simulink model "Shanthan_Heeirthan_EE469S3D_R45 (1)"  (R2023a)
settings: Solver=FixedStepDiscrete  StartTime=0.0  StopTime=120  FixedStep=dt0  RelTol=1e-3  EnableMultiTasking=on
PostLoadFcn:
  | %Set the size for the model
  | set_param(gcs,'Location',[10 10 1270 970])
  | %Set the zoom factor for the model
  | set_param(gcs,'ZoomFactor','100')
InitFcn:
  | tic
  | % Students Add call to their M-file HERE
  | Shanthan_Heeirthan_EE460_Final
  | INIT_S3D_01
StartFcn:
  | tend0=toc;
  | tic;
StopFcn:
  | tend=toc;
  | disp(['Simulation time = ' num2str(tout(end)) ' sec'])
  | disp(['Real time = ' num2str(tend) ' sec'])
  | title('DONE')
  | SCORE=round((max(0,120-tout(end)-tend0))*4+10*(40-FuelBurned)+sum(100*double(PDONE)-100*double(PDONE<.5)));
  | PlotS3D(PlotInput);
  | text(15,22,['S: ' num2str(SCORE)]);
values from neighbouring files (symbols this model uses):
  A = [0 1 0 0 0 0 ... (first row only)    [Shanthan_Heeirthan_EE460_Final (1).m]
  B = [0 0 0 ... (first row only)    [Shanthan_Heeirthan_EE460_Final (1).m]
  bm = [1 1 -1 -1 0 0 0 0; 0 0 0 0 -1 1 1 -1; -1 1 -1 1 3 -3 3 -3]    [Shanthan_Heeirthan_EE460_Final (1).m]
  C = [1 0 0 0 0 0 ... (first row only)    [Shanthan_Heeirthan_EE460_Final (1).m]
  D = [0 0 0 ... (first row only)    [Shanthan_Heeirthan_EE460_Final (1).m]
  Denchptheta = TFchptheta.Den{1}    [Shanthan_Heeirthan_EE460_Final (1).m]
  Denchpxy = TFchpxy.Den{1}    [Shanthan_Heeirthan_EE460_Final (1).m]
  Denclptheta = TFclptheta.Den{1}    [Shanthan_Heeirthan_EE460_Final (1).m]
  Denclpxy = TFclpxy.Den{1}    [Shanthan_Heeirthan_EE460_Final (1).m]
  Denlp = TFlp.Den{1}    [Shanthan_Heeirthan_EE460_Final (1).m]
  Kd = 2.1+0    (= 2.1)    [Shanthan_Heeirthan_EE460_Final (1).m]
  Ki = 0.0001    [Shanthan_Heeirthan_EE460_Final (1).m]
  Kp = 1.1+0.2    (= 1.3)    [Shanthan_Heeirthan_EE460_Final (1).m]
  L = place(A',C',ep)'    [Shanthan_Heeirthan_EE460_Final (1).m]
  Numchptheta = TFchptheta.Num{1}    [Shanthan_Heeirthan_EE460_Final (1).m]
  Numchpxy = TFchpxy.Num{1}    [Shanthan_Heeirthan_EE460_Final (1).m]
  Numclptheta = TFclptheta.Num{1}    [Shanthan_Heeirthan_EE460_Final (1).m]
  Numclpxy = TFclpxy.Num{1}    [Shanthan_Heeirthan_EE460_Final (1).m]
  Numlp = TFlp.Num{1}    [Shanthan_Heeirthan_EE460_Final (1).m]
  Pnewdata = [LVL.P1 LVL.P2 LVL.P3 LVL.P4]    [Shanthan_Heeirthan_EE460_Final (1).m]
  Sconfig = 1    [Shanthan_Heeirthan_EE460_Final (1).m]
  TFP1 = 2    [Shanthan_Heeirthan_EE460_Final (1).m]
  TFP1z = 1    [Shanthan_Heeirthan_EE460_Final (1).m]
  TFP2 = 2    [Shanthan_Heeirthan_EE460_Final (1).m]
  TFP2z = 1    [Shanthan_Heeirthan_EE460_Final (1).m]
  TFP3 = 2    [Shanthan_Heeirthan_EE460_Final (1).m]
  TFP3z = 1    [Shanthan_Heeirthan_EE460_Final (1).m]
  TFP4 = 2    [Shanthan_Heeirthan_EE460_Final (1).m]
  TFP4z = 1    [Shanthan_Heeirthan_EE460_Final (1).m]
  wcf = 2    [Shanthan_Heeirthan_EE460_Final (1).m]
  wcft = 10    [Shanthan_Heeirthan_EE460_Final (1).m]
undefined symbols (not defined in the file or in its folder): d2r, DiscIntNeverNeededParam, dt, dt0, fr, HM_S, HM_U, J, Jbase, JC0, L13, L24, LVL, M, M1, M2, M3, M4, mdti, Pdata, PTvec, r2d, SLIM, SQ, SSF, TOLdata, ULIM
libraries: simulink x85, aerolibanimutils x1, matrix_library x1
(part 3 of 7)

== system Shanthan_Heeirthan_EE469S3D_R45 (1)/S3D_Plant/Sensors/CASE1/Yaccel ==
  X : Inport
  Abs : Abs  SaturateOnIntegerOverflow=off
  Bus Selector3 : BusSelector  OutputSignals=yddt_mps2
  CURRENT : Subsystem  TreatAsAtomicUnit=on
  Compare To Constant : simulink/Logic and Bit Operations/Compare To Constant  relop=<=  const=0.5  OutDataTypeStr=boolean
  Constant1 : Constant  Value=LVL.Sfail(6)  SampleTime=dt0
  Constant2 : Constant  Value=LVL.Sft(6,1)+rand*(LVL.Sft(6,2)-LVL.Sft(6,1))  SampleTime=dt0
  Digital Clock : DigitalClock  SampleTime=dt0
  Gain : Gain  Gain=LVL.SN
  If : If  IfExpression=u1 < -0.5  ElseIfExpressions=u1 > 0.5 & u1 < 1.5
  Logical Operator : Logic  Operator=OR  AllPortsSameDT=off  OutDataTypeStr=boolean
  MAX : Subsystem  TreatAsAtomicUnit=on
  MIN : Subsystem  TreatAsAtomicUnit=on
  Merge : Merge  Inputs=3
  Quantizer : Quantizer  QuantizationInterval=SQ(6)  SampleTime=dt0
  Random Number : RandomNumber  Variance=LVL.SigSense(6)  Seed=6  SampleTime=dt0
  Relational Operator : RelationalOperator  Operator=<  OutDataTypeStr=boolean  InputSameDT=off
  Saturation : Saturate  UpperLimit=SLIM(6,2)  LowerLimit=SLIM(6,1)
  Sum : Sum  Inputs=|++
  Switch : Switch  Criteria=u2 > Threshold  SaturateOnIntegerOverflow=off  InputSameDT=off
  Unit Delay : UnitDelay  SampleTime=dt0  HasFrameUpgradeWarning=on
  yddt1 : Outport
  wires:
  Saturation/1 -> Quantizer/1
  Quantizer/1 -> yddt1/1, Unit Delay/1
  If/1 -> MIN/Action
  If/2 -> MAX/Action
  Switch/1 -> Saturation/1
  Digital Clock/1 -> Relational Operator/1
  If/3 -> CURRENT/Action
  Unit Delay/1 -> CURRENT/1(In1)
  MAX/1(Out1) -> Merge/2
  Constant2/1 -> Relational Operator/2
  X/1 -> Bus Selector3/1
  CURRENT/1(Out1) -> Merge/3
  MIN/1(Out1) -> Merge/1
  Merge/1 -> Switch/3
  Random Number/1 -> Gain/1
  Gain/1 -> Sum/2
  Bus Selector3/1 -> Sum/1  "<yddt_mps2>"
  Sum/1 -> Switch/1
  Relational Operator/1 -> Logical Operator/1
  Logical Operator/1 -> Switch/2
  Constant1/1 -> Abs/1, If/1
  Abs/1 -> Compare To Constant/1
  Compare To Constant/1 -> Logical Operator/2

== system Shanthan_Heeirthan_EE469S3D_R45 (1)/S3D_Plant/Sensors/CASE1/Ypos1 ==
  X : Inport
  Abs : Abs  SaturateOnIntegerOverflow=off
  Bus Selector3 : BusSelector  OutputSignals=y_m
  CURRENT : Subsystem  TreatAsAtomicUnit=on
  Compare To Constant : simulink/Logic and Bit Operations/Compare To Constant  relop=<=  const=0.5  OutDataTypeStr=boolean
  Constant1 : Constant  Value=LVL.Sfail(4)  SampleTime=dt0
  Constant2 : Constant  Value=LVL.Sft(4,1)+rand*(LVL.Sft(4,2)-LVL.Sft(4,1))  SampleTime=dt0
  Digital Clock : DigitalClock  SampleTime=dt0
  Gain : Gain  Gain=LVL.SN
  If : If  IfExpression=u1 < -0.5  ElseIfExpressions=u1 > 0.5 & u1 < 1.5
  Logical Operator : Logic  Operator=OR  AllPortsSameDT=off  OutDataTypeStr=boolean
  MAX : Subsystem  TreatAsAtomicUnit=on
  MIN : Subsystem  TreatAsAtomicUnit=on
  Merge : Merge  Inputs=3
  Quantizer : Quantizer  QuantizationInterval=SQ(4)  SampleTime=dt0
  Random Number : RandomNumber  Variance=LVL.SigSense(4)  Seed=4  SampleTime=dt0
  Relational Operator : RelationalOperator  Operator=<  OutDataTypeStr=boolean  InputSameDT=off
  Saturation : Saturate  UpperLimit=SLIM(4,2)  LowerLimit=SLIM(4,1)
  Sum : Sum  Inputs=|++
  Switch : Switch  Criteria=u2 > Threshold  SaturateOnIntegerOverflow=off  InputSameDT=off
  Unit Delay : UnitDelay  SampleTime=dt0  HasFrameUpgradeWarning=on
  y1 : Outport
  wires:
  Saturation/1 -> Quantizer/1
  Quantizer/1 -> y1/1, Unit Delay/1
  If/1 -> MIN/Action
  If/2 -> MAX/Action
  Switch/1 -> Saturation/1
  Digital Clock/1 -> Relational Operator/1
  If/3 -> CURRENT/Action
  Unit Delay/1 -> CURRENT/1(In1)
  MAX/1(Out1) -> Merge/2
  Constant2/1 -> Relational Operator/2
  X/1 -> Bus Selector3/1
  CURRENT/1(Out1) -> Merge/3
  MIN/1(Out1) -> Merge/1
  Merge/1 -> Switch/3
  Random Number/1 -> Gain/1
  Gain/1 -> Sum/2
  Bus Selector3/1 -> Sum/1  "<y_m>"
  Sum/1 -> Switch/1
  Relational Operator/1 -> Logical Operator/1
  Logical Operator/1 -> Switch/2
  Constant1/1 -> Abs/1, If/1
  Abs/1 -> Compare To Constant/1
  Compare To Constant/1 -> Logical Operator/2

== system Shanthan_Heeirthan_EE469S3D_R45 (1)/S3D_Plant/Sensors/CASE1/Yvel ==
  X : Inport
  Abs : Abs  SaturateOnIntegerOverflow=off
  Bus Selector3 : BusSelector  OutputSignals=ydt_mps
  CURRENT : Subsystem  TreatAsAtomicUnit=on
  Compare To Constant : simulink/Logic and Bit Operations/Compare To Constant  relop=<=  const=0.5  OutDataTypeStr=boolean
  Constant1 : Constant  Value=LVL.Sfail(5)  SampleTime=dt0
  Constant2 : Constant  Value=LVL.Sft(5,1)+rand*(LVL.Sft(5,2)-LVL.Sft(5,1))  SampleTime=dt0
  Digital Clock : DigitalClock  SampleTime=dt0
  Gain : Gain  Gain=LVL.SN
  If : If  IfExpression=u1 < -0.5  ElseIfExpressions=u1 > 0.5 & u1 < 1.5
  Logical Operator : Logic  Operator=OR  AllPortsSameDT=off  OutDataTypeStr=boolean
  MAX : Subsystem  TreatAsAtomicUnit=on
  MIN : Subsystem  TreatAsAtomicUnit=on
  Merge : Merge  Inputs=3
  Quantizer : Quantizer  QuantizationInterval=SQ(5)  SampleTime=dt0
  Random Number : RandomNumber  Variance=LVL.SigSense(5)  Seed=5  SampleTime=dt0
  Relational Operator : RelationalOperator  Operator=<  OutDataTypeStr=boolean  InputSameDT=off
  Saturation : Saturate  UpperLimit=SLIM(5,2)  LowerLimit=SLIM(5,1)
  Sum : Sum  Inputs=|++
  Switch : Switch  Criteria=u2 > Threshold  SaturateOnIntegerOverflow=off  InputSameDT=off
  Unit Delay : UnitDelay  SampleTime=dt0  HasFrameUpgradeWarning=on
  ydt1 : Outport
  wires:
  Saturation/1 -> Quantizer/1
  Quantizer/1 -> Unit Delay/1, ydt1/1
  Compare To Constant/1 -> Logical Operator/2
  Abs/1 -> Compare To Constant/1
  Constant1/1 -> If/1, Abs/1
  Logical Operator/1 -> Switch/2
  Relational Operator/1 -> Logical Operator/1
  Sum/1 -> Switch/1
  Bus Selector3/1 -> Sum/1  "<ydt_mps>"
  Gain/1 -> Sum/2
  Random Number/1 -> Gain/1
  Merge/1 -> Switch/3
  MIN/1(Out1) -> Merge/1
  CURRENT/1(Out1) -> Merge/3
  X/1 -> Bus Selector3/1
  Constant2/1 -> Relational Operator/2
  MAX/1(Out1) -> Merge/2
  Unit Delay/1 -> CURRENT/1(In1)
  If/3 -> CURRENT/Action
  Digital Clock/1 -> Relational Operator/1
  Switch/1 -> Saturation/1
  If/2 -> MAX/Action
  If/1 -> MIN/Action

== system Shanthan_Heeirthan_EE469S3D_R45 (1)/S3D_Plant/Sensors/CASE2/THTpos1 ==
  X : Inport
  Abs : Abs  SaturateOnIntegerOverflow=off
  Bus Selector3 : BusSelector  OutputSignals=tht_rad
  CURRENT : Subsystem  TreatAsAtomicUnit=on
  Compare To Constant : simulink/Logic and Bit Operations/Compare To Constant  relop=<=  const=0.5  OutDataTypeStr=boolean
  Constant1 : Constant  Value=LVL.Sfail(7)  SampleTime=dt0
  Constant2 : Constant  Value=LVL.Sft(7,1)+rand*(LVL.Sft(7,2)-LVL.Sft(7,1))  SampleTime=dt0
  Digital Clock : DigitalClock  SampleTime=dt0
  Gain : Gain  Gain=LVL.SN
  Gain4 : Gain  Gain=r2d
  If : If  IfExpression=u1 < -0.5  ElseIfExpressions=u1 > 0.5 & u1 < 1.5
  Logical Operator : Logic  Operator=OR  AllPortsSameDT=off  OutDataTypeStr=boolean
  MAX : Subsystem  TreatAsAtomicUnit=on
  MIN : Subsystem  TreatAsAtomicUnit=on
  Merge : Merge  Inputs=3
  Quantizer : Quantizer  QuantizationInterval=SQ(7)  SampleTime=dt0
  Random Number : RandomNumber  Variance=LVL.SigSense(7)  Seed=7  SampleTime=dt0
  Relational Operator : RelationalOperator  Operator=<  OutDataTypeStr=boolean  InputSameDT=off
  Saturation : Saturate  UpperLimit=SLIM(7,2)  LowerLimit=SLIM(7,1)
  Sum : Sum  Inputs=|++
  Switch : Switch  Criteria=u2 > Threshold  SaturateOnIntegerOverflow=off  InputSameDT=off
  Unit Delay : UnitDelay  SampleTime=dt0  HasFrameUpgradeWarning=on
  tht1 : Outport
  wires:
  Saturation/1 -> Quantizer/1
  Switch/1 -> Saturation/1
  If/1 -> MIN/Action
  If/2 -> MAX/Action
  Digital Clock/1 -> Relational Operator/1
  If/3 -> CURRENT/Action
  Unit Delay/1 -> CURRENT/1(In1)
  MAX/1(Out1) -> Merge/2
  Constant2/1 -> Relational Operator/2
  X/1 -> Bus Selector3/1
  CURRENT/1(Out1) -> Merge/3
  MIN/1(Out1) -> Merge/1
  Merge/1 -> Switch/3
  Random Number/1 -> Gain/1
  Gain/1 -> Sum/2
  Bus Selector3/1 -> Gain4/1  "<tht_rad>"
  Sum/1 -> Switch/1
  Relational Operator/1 -> Logical Operator/1
  Logical Operator/1 -> Switch/2
  Constant1/1 -> Abs/1, If/1
  Abs/1 -> Compare To Constant/1
  Compare To Constant/1 -> Logical Operator/2
  Gain4/1 -> Sum/1
  Quantizer/1 -> Unit Delay/1, tht1/1

== system Shanthan_Heeirthan_EE469S3D_R45 (1)/S3D_Plant/Sensors/CASE2/THTpos2 ==
  X : Inport
  Abs : Abs  SaturateOnIntegerOverflow=off
  Bus Selector3 : BusSelector  OutputSignals=tht_rad
  CURRENT : Subsystem  TreatAsAtomicUnit=on
  Compare To Constant : simulink/Logic and Bit Operations/Compare To Constant  relop=<=  const=0.5  OutDataTypeStr=boolean
  Constant1 : Constant  Value=LVL.Sfail(8)  SampleTime=dt0
  Constant2 : Constant  Value=LVL.Sft(8,1)+rand*(LVL.Sft(8,2)-LVL.Sft(8,1))  SampleTime=dt0
  Digital Clock : DigitalClock  SampleTime=dt0
  Gain : Gain  Gain=LVL.SN
  Gain4 : Gain  Gain=r2d
  If : If  IfExpression=u1 < -0.5  ElseIfExpressions=u1 > 0.5 & u1 < 1.5
  Logical Operator : Logic  Operator=OR  AllPortsSameDT=off  OutDataTypeStr=boolean
  MAX : Subsystem  TreatAsAtomicUnit=on
  MIN : Subsystem  TreatAsAtomicUnit=on
  Merge : Merge  Inputs=3
  Quantizer : Quantizer  QuantizationInterval=SQ(7)  SampleTime=dt0
  Random Number : RandomNumber  Variance=LVL.SigSense(7)  Seed=8  SampleTime=dt0
  Relational Operator : RelationalOperator  Operator=<  OutDataTypeStr=boolean  InputSameDT=off
  Saturation : Saturate  UpperLimit=SLIM(7,2)  LowerLimit=SLIM(7,1)
  Sum : Sum  Inputs=|++
  Switch : Switch  Criteria=u2 > Threshold  SaturateOnIntegerOverflow=off  InputSameDT=off
  Unit Delay : UnitDelay  SampleTime=dt0  HasFrameUpgradeWarning=on
  tht1 : Outport
  wires:
  Saturation/1 -> Quantizer/1
  Switch/1 -> Saturation/1
  Quantizer/1 -> Unit Delay/1, tht1/1
  Gain4/1 -> Sum/1
  Compare To Constant/1 -> Logical Operator/2
  Abs/1 -> Compare To Constant/1
  Constant1/1 -> If/1, Abs/1
  Logical Operator/1 -> Switch/2
  Relational Operator/1 -> Logical Operator/1
  Sum/1 -> Switch/1
  Bus Selector3/1 -> Gain4/1  "<tht_rad>"
  Gain/1 -> Sum/2
  Random Number/1 -> Gain/1
  Merge/1 -> Switch/3
  MIN/1(Out1) -> Merge/1
  CURRENT/1(Out1) -> Merge/3
  X/1 -> Bus Selector3/1
  Constant2/1 -> Relational Operator/2
  MAX/1(Out1) -> Merge/2
  Unit Delay/1 -> CURRENT/1(In1)
  If/3 -> CURRENT/Action
  Digital Clock/1 -> Relational Operator/1
  If/2 -> MAX/Action
  If/1 -> MIN/Action

== system Shanthan_Heeirthan_EE469S3D_R45 (1)/S3D_Plant/Sensors/CASE2/THTvel ==
  X : Inport
  Abs : Abs  SaturateOnIntegerOverflow=off
  Bus Selector3 : BusSelector  OutputSignals=thtdt_rps
  CURRENT : Subsystem  TreatAsAtomicUnit=on
  Compare To Constant : simulink/Logic and Bit Operations/Compare To Constant  relop=<=  const=0.5  OutDataTypeStr=boolean
  Constant1 : Constant  Value=LVL.Sfail(9)  SampleTime=dt0
  Constant2 : Constant  Value=LVL.Sft(9,1)+rand*(LVL.Sft(9,2)-LVL.Sft(9,1))  SampleTime=dt0
  Digital Clock : DigitalClock  SampleTime=dt0
  Gain : Gain  Gain=LVL.SN
  Gain4 : Gain  Gain=r2d
  If : If  IfExpression=u1 < -0.5  ElseIfExpressions=u1 > 0.5 & u1 < 1.5
  Logical Operator : Logic  Operator=OR  AllPortsSameDT=off  OutDataTypeStr=boolean
  MAX : Subsystem  TreatAsAtomicUnit=on
  MIN : Subsystem  TreatAsAtomicUnit=on
  Merge : Merge  Inputs=3
  Quantizer : Quantizer  QuantizationInterval=SQ(8)  SampleTime=dt0
  Random Number : RandomNumber  Variance=LVL.SigSense(8)  Seed=9  SampleTime=dt0
  Relational Operator : RelationalOperator  Operator=<  OutDataTypeStr=boolean  InputSameDT=off
  Saturation : Saturate  UpperLimit=SLIM(8,2)  LowerLimit=SLIM(8,1)
  Sum : Sum  Inputs=|++
  Switch : Switch  Criteria=u2 > Threshold  SaturateOnIntegerOverflow=off  InputSameDT=off
  Unit Delay : UnitDelay  SampleTime=dt0  HasFrameUpgradeWarning=on
  thtdt1 : Outport
  wires:
  Saturation/1 -> Quantizer/1
  Compare To Constant/1 -> Logical Operator/2
  Abs/1 -> Compare To Constant/1
  Constant1/1 -> If/1, Abs/1
  Logical Operator/1 -> Switch/2
  Relational Operator/1 -> Logical Operator/1
  Sum/1 -> Switch/1
  Bus Selector3/1 -> Gain4/1  "<thtdt_rps>"
  Gain/1 -> Sum/2
  Random Number/1 -> Gain/1
  Merge/1 -> Switch/3
  MIN/1(Out1) -> Merge/1
  CURRENT/1(Out1) -> Merge/3
  X/1 -> Bus Selector3/1
  Constant2/1 -> Relational Operator/2
  MAX/1(Out1) -> Merge/2
  Unit Delay/1 -> CURRENT/1(In1)
  If/3 -> CURRENT/Action
  Digital Clock/1 -> Relational Operator/1
  Switch/1 -> Saturation/1
  If/2 -> MAX/Action
  If/1 -> MIN/Action
  Gain4/1 -> Sum/1
  Quantizer/1 -> Unit Delay/1, thtdt1/1

== system Shanthan_Heeirthan_EE469S3D_R45 (1)/S3D_Plant/Sensors/CASE2/Xpos1 ==
  X : Inport
  Abs : Abs  SaturateOnIntegerOverflow=off
  Bus Selector3 : BusSelector  OutputSignals=x_m
  CURRENT : Subsystem  TreatAsAtomicUnit=on
  Compare To Constant : simulink/Logic and Bit Operations/Compare To Constant  relop=<=  const=0.5  OutDataTypeStr=boolean
  Constant1 : Constant  Value=LVL.Sfail(1)  SampleTime=dt0
  Constant2 : Constant  Value=LVL.Sft(1,1)+rand*(LVL.Sft(1,2)-LVL.Sft(1,1))  SampleTime=dt0
  Digital Clock : DigitalClock  SampleTime=dt0
  Gain : Gain  Gain=LVL.SN
  If : If  IfExpression=u1 < -0.5  ElseIfExpressions=u1 > 0.5 & u1 < 1.5
  Logical Operator : Logic  Operator=OR  AllPortsSameDT=off  OutDataTypeStr=boolean
  MAX : Subsystem  TreatAsAtomicUnit=on
  MIN : Subsystem  TreatAsAtomicUnit=on
  Merge : Merge  Inputs=3
  Quantizer : Quantizer  QuantizationInterval=SQ(1)  SampleTime=dt0
  Random Number : RandomNumber  Variance=LVL.SigSense(1)  Seed=1  SampleTime=dt0
  Relational Operator : RelationalOperator  Operator=<  OutDataTypeStr=boolean  InputSameDT=off
  Saturation : Saturate  UpperLimit=SLIM(1,2)  LowerLimit=SLIM(1,1)
  Sum : Sum  Inputs=|++
  Switch : Switch  Criteria=u2 > Threshold  SaturateOnIntegerOverflow=off  InputSameDT=off
  Unit Delay : UnitDelay  SampleTime=dt0  HasFrameUpgradeWarning=on
  x1 : Outport
  wires:
  Saturation/1 -> Quantizer/1
  If/1 -> MIN/Action
  If/2 -> MAX/Action
  Switch/1 -> Saturation/1
  Digital Clock/1 -> Relational Operator/1
  If/3 -> CURRENT/Action
  Unit Delay/1 -> CURRENT/1(In1)
  MAX/1(Out1) -> Merge/2
  Constant2/1 -> Relational Operator/2
  X/1 -> Bus Selector3/1
  CURRENT/1(Out1) -> Merge/3
  MIN/1(Out1) -> Merge/1
  Merge/1 -> Switch/3
  Random Number/1 -> Gain/1
  Gain/1 -> Sum/2
  Bus Selector3/1 -> Sum/1  "<x_m>"
  Sum/1 -> Switch/1
  Relational Operator/1 -> Logical Operator/1
  Logical Operator/1 -> Switch/2
  Constant1/1 -> Abs/1, If/1
  Abs/1 -> Compare To Constant/1
  Compare To Constant/1 -> Logical Operator/2
  Quantizer/1 -> x1/1, Unit Delay/1

== system Shanthan_Heeirthan_EE469S3D_R45 (1)/S3D_Plant/Sensors/CASE2/Xpos2 ==
  X : Inport
  Abs : Abs  SaturateOnIntegerOverflow=off
  Bus Selector3 : BusSelector  OutputSignals=x_m
  CURRENT : Subsystem  TreatAsAtomicUnit=on
  Compare To Constant : simulink/Logic and Bit Operations/Compare To Constant  relop=<=  const=0.5  OutDataTypeStr=boolean
  Constant1 : Constant  Value=LVL.Sfail(2)  SampleTime=dt0
  Constant2 : Constant  Value=LVL.Sft(2,1)+rand*(LVL.Sft(2,2)-LVL.Sft(2,1))  SampleTime=dt0
  Digital Clock : DigitalClock  SampleTime=dt0
  Gain : Gain  Gain=LVL.SN
  If : If  IfExpression=u1 < -0.5  ElseIfExpressions=u1 > 0.5 & u1 < 1.5
  Logical Operator : Logic  Operator=OR  AllPortsSameDT=off  OutDataTypeStr=boolean
  MAX : Subsystem  TreatAsAtomicUnit=on
  MIN : Subsystem  TreatAsAtomicUnit=on
  Merge : Merge  Inputs=3
  Quantizer : Quantizer  QuantizationInterval=SQ(1)  SampleTime=dt0
  Random Number : RandomNumber  Variance=LVL.SigSense(1)  Seed=2  SampleTime=dt0
  Relational Operator : RelationalOperator  Operator=<  OutDataTypeStr=boolean  InputSameDT=off
  Saturation : Saturate  UpperLimit=SLIM(1,2)  LowerLimit=SLIM(1,1)
  Sum : Sum  Inputs=|++
  Switch : Switch  Criteria=u2 > Threshold  SaturateOnIntegerOverflow=off  InputSameDT=off
  Unit Delay : UnitDelay  SampleTime=dt0  HasFrameUpgradeWarning=on
  x1 : Outport
  wires:
  Saturation/1 -> Quantizer/1
  Quantizer/1 -> Unit Delay/1, x1/1
  Compare To Constant/1 -> Logical Operator/2
  Abs/1 -> Compare To Constant/1
  Constant1/1 -> If/1, Abs/1
  Logical Operator/1 -> Switch/2
  Relational Operator/1 -> Logical Operator/1
  Sum/1 -> Switch/1
  Bus Selector3/1 -> Sum/1  "<x_m>"
  Gain/1 -> Sum/2
  Random Number/1 -> Gain/1
  Merge/1 -> Switch/3
  MIN/1(Out1) -> Merge/1
  CURRENT/1(Out1) -> Merge/3
  X/1 -> Bus Selector3/1
  Constant2/1 -> Relational Operator/2
  MAX/1(Out1) -> Merge/2
  Unit Delay/1 -> CURRENT/1(In1)
  If/3 -> CURRENT/Action
  Digital Clock/1 -> Relational Operator/1
  Switch/1 -> Saturation/1
  If/2 -> MAX/Action
  If/1 -> MIN/Action

== system Shanthan_Heeirthan_EE469S3D_R45 (1)/S3D_Plant/Sensors/CASE2/Xvel ==
  X : Inport
  Abs : Abs  SaturateOnIntegerOverflow=off
  Bus Selector3 : BusSelector  OutputSignals=xdt_mps
  CURRENT : Subsystem  TreatAsAtomicUnit=on
  Compare To Constant : simulink/Logic and Bit Operations/Compare To Constant  relop=<=  const=0.5  OutDataTypeStr=boolean
  Constant1 : Constant  Value=LVL.Sfail(3)  SampleTime=dt0
  Constant2 : Constant  Value=LVL.Sft(3,1)+rand*(LVL.Sft(3,2)-LVL.Sft(3,1))  SampleTime=dt0
  Digital Clock : DigitalClock  SampleTime=dt0
  Gain : Gain  Gain=LVL.SN
  If : If  IfExpression=u1 < -0.5  ElseIfExpressions=u1 > 0.5 & u1 < 1.5
  Logical Operator : Logic  Operator=OR  AllPortsSameDT=off  OutDataTypeStr=boolean
  MAX : Subsystem  TreatAsAtomicUnit=on
  MIN : Subsystem  TreatAsAtomicUnit=on
  Merge : Merge  Inputs=3
  Quantizer : Quantizer  QuantizationInterval=SQ(2)  SampleTime=dt0
  Random Number : RandomNumber  Variance=LVL.SigSense(2)  Seed=3  SampleTime=dt0
  Relational Operator : RelationalOperator  Operator=<  OutDataTypeStr=boolean  InputSameDT=off
  Saturation : Saturate  UpperLimit=SLIM(2,2)  LowerLimit=SLIM(2,1)
  Sum : Sum  Inputs=|++
  Switch : Switch  Criteria=u2 > Threshold  SaturateOnIntegerOverflow=off  InputSameDT=off
  Unit Delay : UnitDelay  SampleTime=dt0  HasFrameUpgradeWarning=on
  xdt1 : Outport
  wires:
  Saturation/1 -> Quantizer/1
  Compare To Constant/1 -> Logical Operator/2
  Abs/1 -> Compare To Constant/1
  Constant1/1 -> If/1, Abs/1
  Logical Operator/1 -> Switch/2
  Relational Operator/1 -> Logical Operator/1
  Sum/1 -> Switch/1
  Bus Selector3/1 -> Sum/1  "<xdt_mps>"
  Gain/1 -> Sum/2
  Random Number/1 -> Gain/1
  Merge/1 -> Switch/3
  MIN/1(Out1) -> Merge/1
  CURRENT/1(Out1) -> Merge/3
  X/1 -> Bus Selector3/1
  Constant2/1 -> Relational Operator/2
  MAX/1(Out1) -> Merge/2
  Unit Delay/1 -> CURRENT/1(In1)
  If/3 -> CURRENT/Action
  Digital Clock/1 -> Relational Operator/1
  Switch/1 -> Saturation/1
  If/2 -> MAX/Action
  If/1 -> MIN/Action
  Quantizer/1 -> Unit Delay/1, xdt1/1

== system Shanthan_Heeirthan_EE469S3D_R45 (1)/S3D_Plant/Sensors/CASE2/Ypos1 ==
  X : Inport
  Abs : Abs  SaturateOnIntegerOverflow=off
  Bus Selector3 : BusSelector  OutputSignals=y_m
  CURRENT : Subsystem  TreatAsAtomicUnit=on
  Compare To Constant : simulink/Logic and Bit Operations/Compare To Constant  relop=<=  const=0.5  OutDataTypeStr=boolean
  Constant1 : Constant  Value=LVL.Sfail(4)  SampleTime=dt0
  Constant2 : Constant  Value=LVL.Sft(4,1)+rand*(LVL.Sft(4,2)-LVL.Sft(4,1))  SampleTime=dt0
  Digital Clock : DigitalClock  SampleTime=dt0
  Gain : Gain  Gain=LVL.SN
  If : If  IfExpression=u1 < -0.5  ElseIfExpressions=u1 > 0.5 & u1 < 1.5
  Logical Operator : Logic  Operator=OR  AllPortsSameDT=off  OutDataTypeStr=boolean
  MAX : Subsystem  TreatAsAtomicUnit=on
  MIN : Subsystem  TreatAsAtomicUnit=on
  Merge : Merge  Inputs=3
  Quantizer : Quantizer  QuantizationInterval=SQ(4)  SampleTime=dt0
  Random Number : RandomNumber  Variance=LVL.SigSense(4)  Seed=4  SampleTime=dt0
  Relational Operator : RelationalOperator  Operator=<  OutDataTypeStr=boolean  InputSameDT=off
  Saturation : Saturate  UpperLimit=SLIM(4,2)  LowerLimit=SLIM(4,1)
  Sum : Sum  Inputs=|++
  Switch : Switch  Criteria=u2 > Threshold  SaturateOnIntegerOverflow=off  InputSameDT=off
  Unit Delay : UnitDelay  SampleTime=dt0  HasFrameUpgradeWarning=on
  y1 : Outport
  wires:
  Saturation/1 -> Quantizer/1
  Compare To Constant/1 -> Logical Operator/2
  Abs/1 -> Compare To Constant/1
  Constant1/1 -> If/1, Abs/1
  Logical Operator/1 -> Switch/2
  Relational Operator/1 -> Logical Operator/1
  Sum/1 -> Switch/1
  Bus Selector3/1 -> Sum/1  "<y_m>"
  Gain/1 -> Sum/2
  Random Number/1 -> Gain/1
  Merge/1 -> Switch/3
  MIN/1(Out1) -> Merge/1
  CURRENT/1(Out1) -> Merge/3
  X/1 -> Bus Selector3/1
  Constant2/1 -> Relational Operator/2
  MAX/1(Out1) -> Merge/2
  Unit Delay/1 -> CURRENT/1(In1)
  If/3 -> CURRENT/Action
  Digital Clock/1 -> Relational Operator/1
  Switch/1 -> Saturation/1
  If/2 -> MAX/Action
  If/1 -> MIN/Action
  Quantizer/1 -> Unit Delay/1, y1/1

== system Shanthan_Heeirthan_EE469S3D_R45 (1)/S3D_Plant/Sensors/CASE2/Ypos2 ==
  X : Inport
  Abs : Abs  SaturateOnIntegerOverflow=off
  Bus Selector3 : BusSelector  OutputSignals=y_m
  CURRENT : Subsystem  TreatAsAtomicUnit=on
  Compare To Constant : simulink/Logic and Bit Operations/Compare To Constant  relop=<=  const=0.5  OutDataTypeStr=boolean
  Constant1 : Constant  Value=LVL.Sfail(5)  SampleTime=dt0
  Constant2 : Constant  Value=LVL.Sft(5,1)+rand*(LVL.Sft(5,2)-LVL.Sft(5,1))  SampleTime=dt0
  Digital Clock : DigitalClock  SampleTime=dt0
  Gain : Gain  Gain=LVL.SN
  If : If  IfExpression=u1 < -0.5  ElseIfExpressions=u1 > 0.5 & u1 < 1.5
  Logical Operator : Logic  Operator=OR  AllPortsSameDT=off  OutDataTypeStr=boolean
  MAX : Subsystem  TreatAsAtomicUnit=on
  MIN : Subsystem  TreatAsAtomicUnit=on
  Merge : Merge  Inputs=3
  Quantizer : Quantizer  QuantizationInterval=SQ(4)  SampleTime=dt0
  Random Number : RandomNumber  Variance=LVL.SigSense(4)  Seed=5  SampleTime=dt0
  Relational Operator : RelationalOperator  Operator=<  OutDataTypeStr=boolean  InputSameDT=off
  Saturation : Saturate  UpperLimit=SLIM(4,2)  LowerLimit=SLIM(4,1)
  Sum : Sum  Inputs=|++
  Switch : Switch  Criteria=u2 > Threshold  SaturateOnIntegerOverflow=off  InputSameDT=off
  Unit Delay : UnitDelay  SampleTime=dt0  HasFrameUpgradeWarning=on
  y1 : Outport
  wires:
  Saturation/1 -> Quantizer/1
  Quantizer/1 -> y1/1, Unit Delay/1
  If/1 -> MIN/Action
  If/2 -> MAX/Action
  Switch/1 -> Saturation/1
  Digital Clock/1 -> Relational Operator/1
  If/3 -> CURRENT/Action
  Unit Delay/1 -> CURRENT/1(In1)
  MAX/1(Out1) -> Merge/2
  Constant2/1 -> Relational Operator/2
  X/1 -> Bus Selector3/1
  CURRENT/1(Out1) -> Merge/3
  MIN/1(Out1) -> Merge/1
  Merge/1 -> Switch/3
  Random Number/1 -> Gain/1
  Gain/1 -> Sum/2
  Bus Selector3/1 -> Sum/1  "<y_m>"
  Sum/1 -> Switch/1
  Relational Operator/1 -> Logical Operator/1
  Logical Operator/1 -> Switch/2
  Constant1/1 -> Abs/1, If/1
  Abs/1 -> Compare To Constant/1
  Compare To Constant/1 -> Logical Operator/2

== system Shanthan_Heeirthan_EE469S3D_R45 (1)/S3D_Plant/Sensors/CASE2/Yvel ==
  X : Inport
  Abs : Abs  SaturateOnIntegerOverflow=off
  Bus Selector3 : BusSelector  OutputSignals=ydt_mps
  CURRENT : Subsystem  TreatAsAtomicUnit=on
  Compare To Constant : simulink/Logic and Bit Operations/Compare To Constant  relop=<=  const=0.5  OutDataTypeStr=boolean
  Constant1 : Constant  Value=LVL.Sfail(6)  SampleTime=dt0
  Constant2 : Constant  Value=LVL.Sft(6,1)+rand*(LVL.Sft(6,2)-LVL.Sft(6,1))  SampleTime=dt0
  Digital Clock : DigitalClock  SampleTime=dt0
  Gain : Gain  Gain=LVL.SN
  If : If  IfExpression=u1 < -0.5  ElseIfExpressions=u1 > 0.5 & u1 < 1.5
  Logical Operator : Logic  Operator=OR  AllPortsSameDT=off  OutDataTypeStr=boolean
  MAX : Subsystem  TreatAsAtomicUnit=on
  MIN : Subsystem  TreatAsAtomicUnit=on
  Merge : Merge  Inputs=3
  Quantizer : Quantizer  QuantizationInterval=SQ(5)  SampleTime=dt0
  Random Number : RandomNumber  Variance=LVL.SigSense(5)  Seed=6  SampleTime=dt0
  Relational Operator : RelationalOperator  Operator=<  OutDataTypeStr=boolean  InputSameDT=off
  Saturation : Saturate  UpperLimit=SLIM(5,2)  LowerLimit=SLIM(5,1)
  Sum : Sum  Inputs=|++
  Switch : Switch  Criteria=u2 > Threshold  SaturateOnIntegerOverflow=off  InputSameDT=off
  Unit Delay : UnitDelay  SampleTime=dt0  HasFrameUpgradeWarning=on
  ydt1 : Outport
  wires:
  Saturation/1 -> Quantizer/1
  If/1 -> MIN/Action
  If/2 -> MAX/Action
  Switch/1 -> Saturation/1
  Digital Clock/1 -> Relational Operator/1
  If/3 -> CURRENT/Action
  Unit Delay/1 -> CURRENT/1(In1)
  MAX/1(Out1) -> Merge/2
  Constant2/1 -> Relational Operator/2
  X/1 -> Bus Selector3/1
  CURRENT/1(Out1) -> Merge/3
  MIN/1(Out1) -> Merge/1
  Merge/1 -> Switch/3
  Random Number/1 -> Gain/1
  Gain/1 -> Sum/2
  Bus Selector3/1 -> Sum/1  "<ydt_mps>"
  Sum/1 -> Switch/1
  Relational Operator/1 -> Logical Operator/1
  Logical Operator/1 -> Switch/2
  Constant1/1 -> Abs/1, If/1
  Abs/1 -> Compare To Constant/1
  Compare To Constant/1 -> Logical Operator/2
  Quantizer/1 -> ydt1/1, Unit Delay/1

== system Shanthan_Heeirthan_EE469S3D_R45 (1)/S3D_Plant/Sensors/CASE3/THTpos1 ==
  X : Inport
  Abs : Abs  SaturateOnIntegerOverflow=off
  Bus Selector3 : BusSelector  OutputSignals=tht_rad
  CURRENT : Subsystem  TreatAsAtomicUnit=on
  Compare To Constant : simulink/Logic and Bit Operations/Compare To Constant  relop=<=  const=0.5  OutDataTypeStr=boolean
  Constant1 : Constant  Value=LVL.Sfail(7)  SampleTime=dt0
  Constant2 : Constant  Value=LVL.Sft(7,1)+rand*(LVL.Sft(7,2)-LVL.Sft(7,1))  SampleTime=dt0
  Digital Clock : DigitalClock  SampleTime=dt0
  Gain : Gain  Gain=LVL.SN
  Gain4 : Gain  Gain=r2d
  If : If  IfExpression=u1 < -0.5  ElseIfExpressions=u1 > 0.5 & u1 < 1.5
  Logical Operator : Logic  Operator=OR  AllPortsSameDT=off  OutDataTypeStr=boolean
  MAX : Subsystem  TreatAsAtomicUnit=on
  MIN : Subsystem  TreatAsAtomicUnit=on
  Merge : Merge  Inputs=3
  Quantizer : Quantizer  QuantizationInterval=SQ(7)  SampleTime=dt0
  Random Number : RandomNumber  Variance=LVL.SigSense(7)  Seed=7  SampleTime=dt0
  Relational Operator : RelationalOperator  Operator=<  OutDataTypeStr=boolean  InputSameDT=off
  Saturation : Saturate  UpperLimit=SLIM(7,2)  LowerLimit=SLIM(7,1)
  Sum : Sum  Inputs=|++
  Switch : Switch  Criteria=u2 > Threshold  SaturateOnIntegerOverflow=off  InputSameDT=off
  Unit Delay : UnitDelay  SampleTime=dt0  HasFrameUpgradeWarning=on
  tht1 : Outport
  wires:
  Saturation/1 -> Quantizer/1
  Switch/1 -> Saturation/1
  Quantizer/1 -> Unit Delay/1, tht1/1
  Gain4/1 -> Sum/1
  Compare To Constant/1 -> Logical Operator/2
  Abs/1 -> Compare To Constant/1
  Constant1/1 -> If/1, Abs/1
  Logical Operator/1 -> Switch/2
  Relational Operator/1 -> Logical Operator/1
  Sum/1 -> Switch/1
  Bus Selector3/1 -> Gain4/1  "<tht_rad>"
  Gain/1 -> Sum/2
  Random Number/1 -> Gain/1
  Merge/1 -> Switch/3
  MIN/1(Out1) -> Merge/1
  CURRENT/1(Out1) -> Merge/3
  X/1 -> Bus Selector3/1
  Constant2/1 -> Relational Operator/2
  MAX/1(Out1) -> Merge/2
  Unit Delay/1 -> CURRENT/1(In1)
  If/3 -> CURRENT/Action
  Digital Clock/1 -> Relational Operator/1
  If/2 -> MAX/Action
  If/1 -> MIN/Action

== system Shanthan_Heeirthan_EE469S3D_R45 (1)/S3D_Plant/Sensors/CASE3/THTpos2 ==
  X : Inport
  Abs : Abs  SaturateOnIntegerOverflow=off
  Bus Selector3 : BusSelector  OutputSignals=tht_rad
  CURRENT : Subsystem  TreatAsAtomicUnit=on
  Compare To Constant : simulink/Logic and Bit Operations/Compare To Constant  relop=<=  const=0.5  OutDataTypeStr=boolean
  Constant1 : Constant  Value=LVL.Sfail(8)  SampleTime=dt0
  Constant2 : Constant  Value=LVL.Sft(8,1)+rand*(LVL.Sft(8,2)-LVL.Sft(8,1))  SampleTime=dt0
  Digital Clock : DigitalClock  SampleTime=dt0
  Gain : Gain  Gain=LVL.SN
  Gain4 : Gain  Gain=r2d
  If : If  IfExpression=u1 < -0.5  ElseIfExpressions=u1 > 0.5 & u1 < 1.5
  Logical Operator : Logic  Operator=OR  AllPortsSameDT=off  OutDataTypeStr=boolean
  MAX : Subsystem  TreatAsAtomicUnit=on
  MIN : Subsystem  TreatAsAtomicUnit=on
  Merge : Merge  Inputs=3
  Quantizer : Quantizer  QuantizationInterval=SQ(7)  SampleTime=dt0
  Random Number : RandomNumber  Variance=LVL.SigSense(7)  Seed=8  SampleTime=dt0
  Relational Operator : RelationalOperator  Operator=<  OutDataTypeStr=boolean  InputSameDT=off
  Saturation : Saturate  UpperLimit=SLIM(7,2)  LowerLimit=SLIM(7,1)
  Sum : Sum  Inputs=|++
  Switch : Switch  Criteria=u2 > Threshold  SaturateOnIntegerOverflow=off  InputSameDT=off
  Unit Delay : UnitDelay  SampleTime=dt0  HasFrameUpgradeWarning=on
  tht1 : Outport
  wires:
  Saturation/1 -> Quantizer/1
  If/1 -> MIN/Action
  If/2 -> MAX/Action
  Digital Clock/1 -> Relational Operator/1
  If/3 -> CURRENT/Action
  Unit Delay/1 -> CURRENT/1(In1)
  MAX/1(Out1) -> Merge/2
  Constant2/1 -> Relational Operator/2
  X/1 -> Bus Selector3/1
  CURRENT/1(Out1) -> Merge/3
  MIN/1(Out1) -> Merge/1
  Merge/1 -> Switch/3
  Random Number/1 -> Gain/1
  Gain/1 -> Sum/2
  Bus Selector3/1 -> Gain4/1  "<tht_rad>"
  Sum/1 -> Switch/1
  Relational Operator/1 -> Logical Operator/1
  Logical Operator/1 -> Switch/2
  Constant1/1 -> Abs/1, If/1
  Abs/1 -> Compare To Constant/1
  Compare To Constant/1 -> Logical Operator/2
  Gain4/1 -> Sum/1
  Switch/1 -> Saturation/1
  Quantizer/1 -> Unit Delay/1, tht1/1

== system Shanthan_Heeirthan_EE469S3D_R45 (1)/S3D_Plant/Sensors/CASE3/THTpos3 ==
  X : Inport
  Abs : Abs  SaturateOnIntegerOverflow=off
  Bus Selector3 : BusSelector  OutputSignals=tht_rad
  CURRENT : Subsystem  TreatAsAtomicUnit=on
  Compare To Constant : simulink/Logic and Bit Operations/Compare To Constant  relop=<=  const=0.5  OutDataTypeStr=boolean
  Constant1 : Constant  Value=LVL.Sfail(9)  SampleTime=dt0
  Constant2 : Constant  Value=LVL.Sft(9,1)+rand*(LVL.Sft(9,2)-LVL.Sft(9,1))  SampleTime=dt0
  Digital Clock : DigitalClock  SampleTime=dt0
  Gain : Gain  Gain=LVL.SN
  Gain4 : Gain  Gain=r2d
  If : If  IfExpression=u1 < -0.5  ElseIfExpressions=u1 > 0.5 & u1 < 1.5
  Logical Operator : Logic  Operator=OR  AllPortsSameDT=off  OutDataTypeStr=boolean
  MAX : Subsystem  TreatAsAtomicUnit=on
  MIN : Subsystem  TreatAsAtomicUnit=on
  Merge : Merge  Inputs=3
  Quantizer : Quantizer  QuantizationInterval=SQ(7)  SampleTime=dt0
  Random Number : RandomNumber  Variance=LVL.SigSense(7)  Seed=9  SampleTime=dt0
  Relational Operator : RelationalOperator  Operator=<  OutDataTypeStr=boolean  InputSameDT=off
  Saturation : Saturate  UpperLimit=SLIM(7,2)  LowerLimit=SLIM(7,1)
  Sum : Sum  Inputs=|++
  Switch : Switch  Criteria=u2 > Threshold  SaturateOnIntegerOverflow=off  InputSameDT=off
  Unit Delay : UnitDelay  SampleTime=dt0  HasFrameUpgradeWarning=on
  tht1 : Outport
  wires:
  Saturation/1 -> Quantizer/1
  Switch/1 -> Saturation/1
  Quantizer/1 -> Unit Delay/1, tht1/1
  Gain4/1 -> Sum/1
  Compare To Constant/1 -> Logical Operator/2
  Abs/1 -> Compare To Constant/1
  Constant1/1 -> If/1, Abs/1
  Logical Operator/1 -> Switch/2
  Relational Operator/1 -> Logical Operator/1
  Sum/1 -> Switch/1
  Bus Selector3/1 -> Gain4/1  "<tht_rad>"
  Gain/1 -> Sum/2
  Random Number/1 -> Gain/1
  Merge/1 -> Switch/3
  MIN/1(Out1) -> Merge/1
  CURRENT/1(Out1) -> Merge/3
  X/1 -> Bus Selector3/1
  Constant2/1 -> Relational Operator/2
  MAX/1(Out1) -> Merge/2
  Unit Delay/1 -> CURRENT/1(In1)
  If/3 -> CURRENT/Action
  Digital Clock/1 -> Relational Operator/1
  If/2 -> MAX/Action
  If/1 -> MIN/Action

== system Shanthan_Heeirthan_EE469S3D_R45 (1)/S3D_Plant/Sensors/CASE3/Xpos1 ==
  X : Inport
  Abs : Abs  SaturateOnIntegerOverflow=off
  Bus Selector3 : BusSelector  OutputSignals=x_m
  CURRENT : Subsystem  TreatAsAtomicUnit=on
  Compare To Constant : simulink/Logic and Bit Operations/Compare To Constant  relop=<=  const=0.5  OutDataTypeStr=boolean
  Constant1 : Constant  Value=LVL.Sfail(1)  SampleTime=dt0
  Constant2 : Constant  Value=LVL.Sft(1,1)+rand*(LVL.Sft(1,2)-LVL.Sft(1,1))  SampleTime=dt0
  Digital Clock : DigitalClock  SampleTime=dt0
  Gain : Gain  Gain=LVL.SN
  If : If  IfExpression=u1 < -0.5  ElseIfExpressions=u1 > 0.5 & u1 < 1.5
  Logical Operator : Logic  Operator=OR  AllPortsSameDT=off  OutDataTypeStr=boolean
  MAX : Subsystem  TreatAsAtomicUnit=on
  MIN : Subsystem  TreatAsAtomicUnit=on
  Merge : Merge  Inputs=3
  Quantizer : Quantizer  QuantizationInterval=SQ(1)  SampleTime=dt0
  Random Number : RandomNumber  Variance=LVL.SigSense(1)  Seed=1  SampleTime=dt0
  Relational Operator : RelationalOperator  Operator=<  OutDataTypeStr=boolean  InputSameDT=off
  Saturation : Saturate  UpperLimit=SLIM(1,2)  LowerLimit=SLIM(1,1)
  Sum : Sum  Inputs=|++
  Switch : Switch  Criteria=u2 > Threshold  SaturateOnIntegerOverflow=off  InputSameDT=off
  Unit Delay : UnitDelay  SampleTime=dt0  HasFrameUpgradeWarning=on
  x1 : Outport
  wires:
  Saturation/1 -> Quantizer/1
  Quantizer/1 -> Unit Delay/1, x1/1
  Compare To Constant/1 -> Logical Operator/2
  Abs/1 -> Compare To Constant/1
  Constant1/1 -> If/1, Abs/1
  Logical Operator/1 -> Switch/2
  Relational Operator/1 -> Logical Operator/1
  Sum/1 -> Switch/1
  Bus Selector3/1 -> Sum/1  "<x_m>"
  Gain/1 -> Sum/2
  Random Number/1 -> Gain/1
  Merge/1 -> Switch/3
  MIN/1(Out1) -> Merge/1
  CURRENT/1(Out1) -> Merge/3
  X/1 -> Bus Selector3/1
  Constant2/1 -> Relational Operator/2
  MAX/1(Out1) -> Merge/2
  Unit Delay/1 -> CURRENT/1(In1)
  If/3 -> CURRENT/Action
  Digital Clock/1 -> Relational Operator/1
  Switch/1 -> Saturation/1
  If/2 -> MAX/Action
  If/1 -> MIN/Action

== system Shanthan_Heeirthan_EE469S3D_R45 (1)/S3D_Plant/Sensors/CASE3/Xpos2 ==
  X : Inport
  Abs : Abs  SaturateOnIntegerOverflow=off
  Bus Selector3 : BusSelector  OutputSignals=x_m
  CURRENT : Subsystem  TreatAsAtomicUnit=on
  Compare To Constant : simulink/Logic and Bit Operations/Compare To Constant  relop=<=  const=0.5  OutDataTypeStr=boolean
  Constant1 : Constant  Value=LVL.Sfail(2)  SampleTime=dt0
  Constant2 : Constant  Value=LVL.Sft(2,1)+rand*(LVL.Sft(2,2)-LVL.Sft(2,1))  SampleTime=dt0
  Digital Clock : DigitalClock  SampleTime=dt0
  Gain : Gain  Gain=LVL.SN
  If : If  IfExpression=u1 < -0.5  ElseIfExpressions=u1 > 0.5 & u1 < 1.5
  Logical Operator : Logic  Operator=OR  AllPortsSameDT=off  OutDataTypeStr=boolean
  MAX : Subsystem  TreatAsAtomicUnit=on
  MIN : Subsystem  TreatAsAtomicUnit=on
  Merge : Merge  Inputs=3
  Quantizer : Quantizer  QuantizationInterval=SQ(1)  SampleTime=dt0
  Random Number : RandomNumber  Variance=LVL.SigSense(1)  Seed=2  SampleTime=dt0
  Relational Operator : RelationalOperator  Operator=<  OutDataTypeStr=boolean  InputSameDT=off
  Saturation : Saturate  UpperLimit=SLIM(1,2)  LowerLimit=SLIM(1,1)
  Sum : Sum  Inputs=|++
  Switch : Switch  Criteria=u2 > Threshold  SaturateOnIntegerOverflow=off  InputSameDT=off
  Unit Delay : UnitDelay  SampleTime=dt0  HasFrameUpgradeWarning=on
  xdt1 : Outport
  wires:
  Saturation/1 -> Quantizer/1
  Quantizer/1 -> xdt1/1, Unit Delay/1
  If/1 -> MIN/Action
  If/2 -> MAX/Action
  Switch/1 -> Saturation/1
  Digital Clock/1 -> Relational Operator/1
  If/3 -> CURRENT/Action
  Unit Delay/1 -> CURRENT/1(In1)
  MAX/1(Out1) -> Merge/2
  Constant2/1 -> Relational Operator/2
  X/1 -> Bus Selector3/1
  CURRENT/1(Out1) -> Merge/3
  MIN/1(Out1) -> Merge/1
  Merge/1 -> Switch/3
  Random Number/1 -> Gain/1
  Gain/1 -> Sum/2
  Bus Selector3/1 -> Sum/1  "<x_m>"
  Sum/1 -> Switch/1
  Relational Operator/1 -> Logical Operator/1
  Logical Operator/1 -> Switch/2
  Constant1/1 -> Abs/1, If/1
  Abs/1 -> Compare To Constant/1
  Compare To Constant/1 -> Logical Operator/2

== system Shanthan_Heeirthan_EE469S3D_R45 (1)/S3D_Plant/Sensors/CASE3/Xpos3 ==
  X : Inport
  Abs : Abs  SaturateOnIntegerOverflow=off
  Bus Selector3 : BusSelector  OutputSignals=x_m
  CURRENT : Subsystem  TreatAsAtomicUnit=on
  Compare To Constant : simulink/Logic and Bit Operations/Compare To Constant  relop=<=  const=0.5  OutDataTypeStr=boolean
  Constant1 : Constant  Value=LVL.Sfail(3)  SampleTime=dt0
  Constant2 : Constant  Value=LVL.Sft(3,1)+rand*(LVL.Sft(3,2)-LVL.Sft(3,1))  SampleTime=dt0
  Digital Clock : DigitalClock  SampleTime=dt0
  Gain : Gain  Gain=LVL.SN
  If : If  IfExpression=u1 < -0.5  ElseIfExpressions=u1 > 0.5 & u1 < 1.5
  Logical Operator : Logic  Operator=OR  AllPortsSameDT=off  OutDataTypeStr=boolean
  MAX : Subsystem  TreatAsAtomicUnit=on
  MIN : Subsystem  TreatAsAtomicUnit=on
  Merge : Merge  Inputs=3
  Quantizer : Quantizer  QuantizationInterval=SQ(1)  SampleTime=dt0
  Random Number : RandomNumber  Variance=LVL.SigSense(1)  Seed=3  SampleTime=dt0
  Relational Operator : RelationalOperator  Operator=<  OutDataTypeStr=boolean  InputSameDT=off
  Saturation : Saturate  UpperLimit=SLIM(1,2)  LowerLimit=SLIM(1,1)
  Sum : Sum  Inputs=|++
  Switch : Switch  Criteria=u2 > Threshold  SaturateOnIntegerOverflow=off  InputSameDT=off
  Unit Delay : UnitDelay  SampleTime=dt0  HasFrameUpgradeWarning=on
  xddt1 : Outport
  wires:
  Saturation/1 -> Quantizer/1
  Quantizer/1 -> Unit Delay/1, xddt1/1
  Compare To Constant/1 -> Logical Operator/2
  Abs/1 -> Compare To Constant/1
  Constant1/1 -> If/1, Abs/1
  Logical Operator/1 -> Switch/2
  Relational Operator/1 -> Logical Operator/1
  Sum/1 -> Switch/1
  Bus Selector3/1 -> Sum/1  "<x_m>"
  Gain/1 -> Sum/2
  Random Number/1 -> Gain/1
  Merge/1 -> Switch/3
  MIN/1(Out1) -> Merge/1
  CURRENT/1(Out1) -> Merge/3
  X/1 -> Bus Selector3/1
  Constant2/1 -> Relational Operator/2
  MAX/1(Out1) -> Merge/2
  Unit Delay/1 -> CURRENT/1(In1)
  If/3 -> CURRENT/Action
  Digital Clock/1 -> Relational Operator/1
  Switch/1 -> Saturation/1
  If/2 -> MAX/Action
  If/1 -> MIN/Action

== system Shanthan_Heeirthan_EE469S3D_R45 (1)/S3D_Plant/Sensors/CASE3/Ypos1 ==
  X : Inport
  Abs : Abs  SaturateOnIntegerOverflow=off
  Bus Selector3 : BusSelector  OutputSignals=y_m
  CURRENT : Subsystem  TreatAsAtomicUnit=on
  Compare To Constant : simulink/Logic and Bit Operations/Compare To Constant  relop=<=  const=0.5  OutDataTypeStr=boolean
  Constant1 : Constant  Value=LVL.Sfail(4)  SampleTime=dt0
  Constant2 : Constant  Value=LVL.Sft(4,1)+rand*(LVL.Sft(4,2)-LVL.Sft(4,1))  SampleTime=dt0
  Digital Clock : DigitalClock  SampleTime=dt0
  Gain : Gain  Gain=LVL.SN
  If : If  IfExpression=u1 < -0.5  ElseIfExpressions=u1 > 0.5 & u1 < 1.5
  Logical Operator : Logic  Operator=OR  AllPortsSameDT=off  OutDataTypeStr=boolean
  MAX : Subsystem  TreatAsAtomicUnit=on
  MIN : Subsystem  TreatAsAtomicUnit=on
  Merge : Merge  Inputs=3
  Quantizer : Quantizer  QuantizationInterval=SQ(4)  SampleTime=dt0
  Random Number : RandomNumber  Variance=LVL.SigSense(4)  Seed=4  SampleTime=dt0
  Relational Operator : RelationalOperator  Operator=<  OutDataTypeStr=boolean  InputSameDT=off
  Saturation : Saturate  UpperLimit=SLIM(4,2)  LowerLimit=SLIM(4,1)
  Sum : Sum  Inputs=|++
  Switch : Switch  Criteria=u2 > Threshold  SaturateOnIntegerOverflow=off  InputSameDT=off
  Unit Delay : UnitDelay  SampleTime=dt0  HasFrameUpgradeWarning=on
  y1 : Outport
  wires:
  Saturation/1 -> Quantizer/1
  Quantizer/1 -> y1/1, Unit Delay/1
  If/1 -> MIN/Action
  If/2 -> MAX/Action
  Switch/1 -> Saturation/1
  Digital Clock/1 -> Relational Operator/1
  If/3 -> CURRENT/Action
  Unit Delay/1 -> CURRENT/1(In1)
  MAX/1(Out1) -> Merge/2
  Constant2/1 -> Relational Operator/2
  X/1 -> Bus Selector3/1
  CURRENT/1(Out1) -> Merge/3
  MIN/1(Out1) -> Merge/1
  Merge/1 -> Switch/3
  Random Number/1 -> Gain/1
  Gain/1 -> Sum/2
  Bus Selector3/1 -> Sum/1  "<y_m>"
  Sum/1 -> Switch/1
  Relational Operator/1 -> Logical Operator/1
  Logical Operator/1 -> Switch/2
  Constant1/1 -> Abs/1, If/1
  Abs/1 -> Compare To Constant/1
  Compare To Constant/1 -> Logical Operator/2

== system Shanthan_Heeirthan_EE469S3D_R45 (1)/S3D_Plant/Sensors/CASE3/Ypos2 ==
  X : Inport
  Abs : Abs  SaturateOnIntegerOverflow=off
  Bus Selector3 : BusSelector  OutputSignals=y_m
  CURRENT : Subsystem  TreatAsAtomicUnit=on
  Compare To Constant : simulink/Logic and Bit Operations/Compare To Constant  relop=<=  const=0.5  OutDataTypeStr=boolean
  Constant1 : Constant  Value=LVL.Sfail(5)  SampleTime=dt0
  Constant2 : Constant  Value=LVL.Sft(5,1)+rand*(LVL.Sft(5,2)-LVL.Sft(5,1))  SampleTime=dt0
  Digital Clock : DigitalClock  SampleTime=dt0
  Gain : Gain  Gain=LVL.SN
  If : If  IfExpression=u1 < -0.5  ElseIfExpressions=u1 > 0.5 & u1 < 1.5
  Logical Operator : Logic  Operator=OR  AllPortsSameDT=off  OutDataTypeStr=boolean
  MAX : Subsystem  TreatAsAtomicUnit=on
  MIN : Subsystem  TreatAsAtomicUnit=on
  Merge : Merge  Inputs=3
  Quantizer : Quantizer  QuantizationInterval=SQ(4)  SampleTime=dt0
  Random Number : RandomNumber  Variance=LVL.SigSense(4)  Seed=5  SampleTime=dt0
  Relational Operator : RelationalOperator  Operator=<  OutDataTypeStr=boolean  InputSameDT=off
  Saturation : Saturate  UpperLimit=SLIM(4,2)  LowerLimit=SLIM(4,1)
  Sum : Sum  Inputs=|++
  Switch : Switch  Criteria=u2 > Threshold  SaturateOnIntegerOverflow=off  InputSameDT=off
  Unit Delay : UnitDelay  SampleTime=dt0  HasFrameUpgradeWarning=on
  y1 : Outport
  wires:
  Saturation/1 -> Quantizer/1
  Compare To Constant/1 -> Logical Operator/2
  Abs/1 -> Compare To Constant/1
  Constant1/1 -> If/1, Abs/1
  Logical Operator/1 -> Switch/2
  Relational Operator/1 -> Logical Operator/1
  Sum/1 -> Switch/1
  Bus Selector3/1 -> Sum/1  "<y_m>"
  Gain/1 -> Sum/2
  Random Number/1 -> Gain/1
  Merge/1 -> Switch/3
  MIN/1(Out1) -> Merge/1
  CURRENT/1(Out1) -> Merge/3
  X/1 -> Bus Selector3/1
  Constant2/1 -> Relational Operator/2
  MAX/1(Out1) -> Merge/2
  Unit Delay/1 -> CURRENT/1(In1)
  If/3 -> CURRENT/Action
  Digital Clock/1 -> Relational Operator/1
  Switch/1 -> Saturation/1
  If/2 -> MAX/Action
  If/1 -> MIN/Action
  Quantizer/1 -> Unit Delay/1, y1/1

== system Shanthan_Heeirthan_EE469S3D_R45 (1)/S3D_Plant/Sensors/CASE3/Ypos3 ==
  X : Inport
  Abs : Abs  SaturateOnIntegerOverflow=off
  Bus Selector3 : BusSelector  OutputSignals=y_m
  CURRENT : Subsystem  TreatAsAtomicUnit=on
  Compare To Constant : simulink/Logic and Bit Operations/Compare To Constant  relop=<=  const=0.5  OutDataTypeStr=boolean
  Constant1 : Constant  Value=LVL.Sfail(6)  SampleTime=dt0
  Constant2 : Constant  Value=LVL.Sft(6,1)+rand*(LVL.Sft(6,2)-LVL.Sft(6,1))  SampleTime=dt0
  Digital Clock : DigitalClock  SampleTime=dt0
  Gain : Gain  Gain=LVL.SN
  If : If  IfExpression=u1 < -0.5  ElseIfExpressions=u1 > 0.5 & u1 < 1.5
  Logical Operator : Logic  Operator=OR  AllPortsSameDT=off  OutDataTypeStr=boolean
  MAX : Subsystem  TreatAsAtomicUnit=on
  MIN : Subsystem  TreatAsAtomicUnit=on
  Merge : Merge  Inputs=3
  Quantizer : Quantizer  QuantizationInterval=SQ(4)  SampleTime=dt0
  Random Number : RandomNumber  Variance=LVL.SigSense(4)  Seed=6  SampleTime=dt0
  Relational Operator : RelationalOperator  Operator=<  OutDataTypeStr=boolean  InputSameDT=off
  Saturation : Saturate  UpperLimit=SLIM(4,2)  LowerLimit=SLIM(4,1)
  Sum : Sum  Inputs=|++
  Switch : Switch  Criteria=u2 > Threshold  SaturateOnIntegerOverflow=off  InputSameDT=off
  Unit Delay : UnitDelay  SampleTime=dt0  HasFrameUpgradeWarning=on
  y1 : Outport
  wires:
  Saturation/1 -> Quantizer/1
  Quantizer/1 -> y1/1, Unit Delay/1
  If/1 -> MIN/Action
  If/2 -> MAX/Action
  Switch/1 -> Saturation/1
  Digital Clock/1 -> Relational Operator/1
  If/3 -> CURRENT/Action
  Unit Delay/1 -> CURRENT/1(In1)
  MAX/1(Out1) -> Merge/2
  Constant2/1 -> Relational Operator/2
  X/1 -> Bus Selector3/1
  CURRENT/1(Out1) -> Merge/3
  MIN/1(Out1) -> Merge/1
  Merge/1 -> Switch/3
  Random Number/1 -> Gain/1
  Gain/1 -> Sum/2
  Bus Selector3/1 -> Sum/1  "<y_m>"
  Sum/1 -> Switch/1
  Relational Operator/1 -> Logical Operator/1
  Logical Operator/1 -> Switch/2
  Constant1/1 -> Abs/1, If/1
  Abs/1 -> Compare To Constant/1
  Compare To Constant/1 -> Logical Operator/2

== system Shanthan_Heeirthan_EE469S3D_R45 (1)/S3D_Plant/Sensors/HealthMonitoring/Subsystem ==
  In1 : Inport
  Compare To Constant : simulink/Logic and Bit Operations/Compare To Constant  relop=>=  const=HM_S  OutDataTypeStr=boolean
  Constant : Constant  Value=0
  Constant1 : Constant
  Logical Operator : Logic  Operator=OR  AllPortsSameDT=off  OutDataTypeStr=boolean
  Sum : Sum  Inputs=|+-  OutDataTypeStr=int32
  Sum1 : Sum  Inputs=|++
  Switch : Switch  Criteria=u2 > Threshold  Threshold=eps  SaturateOnIntegerOverflow=off  InputSameDT=off
  Unit Delay : UnitDelay  SampleTime=dt0  HasFrameUpgradeWarning=on
  Unit Delay1 : UnitDelay  SampleTime=dt0  HasFrameUpgradeWarning=on
  Unit Delay2 : UnitDelay  SampleTime=dt0  HasFrameUpgradeWarning=on
  Out1 : Outport
  wires:
  Logical Operator/1 -> Unit Delay2/1, Out1/1
  Constant1/1 -> Sum1/1
  Compare To Constant/1 -> Logical Operator/1
  Switch/1 -> Unit Delay1/1, Compare To Constant/1
  In1/1 -> Sum/1, Unit Delay/1
  Unit Delay2/1 -> Logical Operator/2
  Unit Delay/1 -> Sum/2
  Sum/1 -> Switch/2
  Sum1/1 -> Switch/3
  Unit Delay1/1 -> Sum1/2
  Constant/1 -> Switch/1

== system Shanthan_Heeirthan_EE469S3D_R45 (1)/S3D_Plant/Sensors/HealthMonitoring/Subsystem1 ==
  In1 : Inport
  Compare To Constant : simulink/Logic and Bit Operations/Compare To Constant  relop=>=  const=HM_S  OutDataTypeStr=boolean
  Constant : Constant  Value=0
  Constant1 : Constant
  Logical Operator : Logic  Operator=OR  AllPortsSameDT=off  OutDataTypeStr=boolean
  Sum : Sum  Inputs=|+-  OutDataTypeStr=int32
  Sum1 : Sum  Inputs=|++
  Switch : Switch  Criteria=u2 > Threshold  Threshold=eps  SaturateOnIntegerOverflow=off  InputSameDT=off
  Unit Delay : UnitDelay  SampleTime=dt0  HasFrameUpgradeWarning=on
  Unit Delay1 : UnitDelay  SampleTime=dt0  HasFrameUpgradeWarning=on
  Unit Delay2 : UnitDelay  SampleTime=dt0  HasFrameUpgradeWarning=on
  Out1 : Outport
  wires:
  Constant/1 -> Switch/1
  Unit Delay1/1 -> Sum1/2
  Sum1/1 -> Switch/3
  Sum/1 -> Switch/2
  Unit Delay/1 -> Sum/2
  Unit Delay2/1 -> Logical Operator/2
  In1/1 -> Unit Delay/1, Sum/1
  Switch/1 -> Compare To Constant/1, Unit Delay1/1
  Compare To Constant/1 -> Logical Operator/1
  Constant1/1 -> Sum1/1
  Logical Operator/1 -> Out1/1, Unit Delay2/1
